simulink model "Group44PACEMAKER"  (R2022b)
settings: Solver=FixedStepAuto  StartTime=0.0  StopTime=4  FixedStep=1e-3  RelTol=1e-3  EnableMultiTasking=on
undefined symbols (not defined in the file): D0, D1, D10, D11, D12, D13, D2, D3, D4, D5, D6, D7, D8, D9, PTA0, PTA1, PTA2, PTB23, PTB9, PTC16, PTC17, PTC2, PTC3, PTC4, PTD0, PTD1, PTD2, PTD3
libraries: frdmk64flib x14
settings Model: PacingRate=0.200000  ExtModeTrigDuration=5  LastModifiedBy=Admin
settings OptimizationCC: EnhancedBackFolding=on  PassReuseOutputArgsAs=Individual arguments  ZeroExternalMemoryAtStartup=off  ZeroInternalMemoryAtStartup=off  MaxStackSize=64  OptimizeBlockOrder=speed  DifferentSizesBufferReuse=on  OptimizationCustomize=off  EfficientTunableParamExpr=on
settings DebuggingCC: ParameterTunabilityLossMsg=error
settings HardwareCC: ProdBitPerPointer=32  ProdBitPerSizeT=32  ProdBitPerPtrDiffT=32  ProdLargestAtomicInteger=Long  ProdLargestAtomicFloat=Double  ProdWordSize=32  ProdHWDeviceType=ARM Compatible->ARM Cortex
settings SFSimCC: MATLABDynamicMemAlloc=off
settings RTWCC: Description=Embedded Coder  SystemTargetFile=ert.tlc  HardwareBoard=NXP FRDM-K64F  TLCOptions="-aInlineSetEventsForThisBaseRateFcn=TLC_FALSE -aSuppressMultiTaskScheduler=TLC_FALSE  -aRateBasedStepFcn=0"  TemplateMakefile=ert_default_tmf  Toolchain=GNU Tools for ARM Embedded Processors
settings CodeAppCC: ForceParamTrailComments=on  IgnoreCustomStorageClasses=off  OperatorAnnotations=on  SimulinkDataObjDesc=on  SFDataObjDesc=on  InsertBlockDesc=on
settings ERTTargetCC: ExtModeTransport=4  ExtModeMexFile=sendToCommService

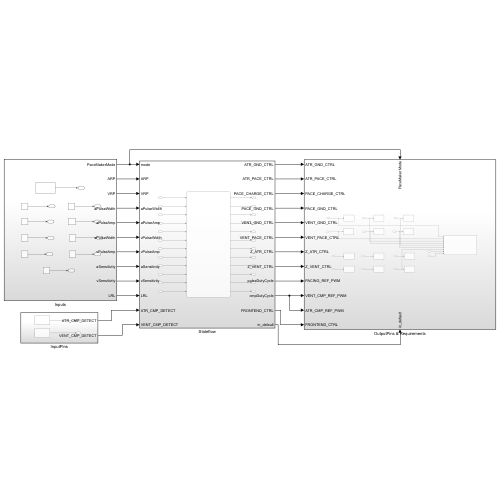
[thumbnail: Simulink's stored preview of the top-level diagram]
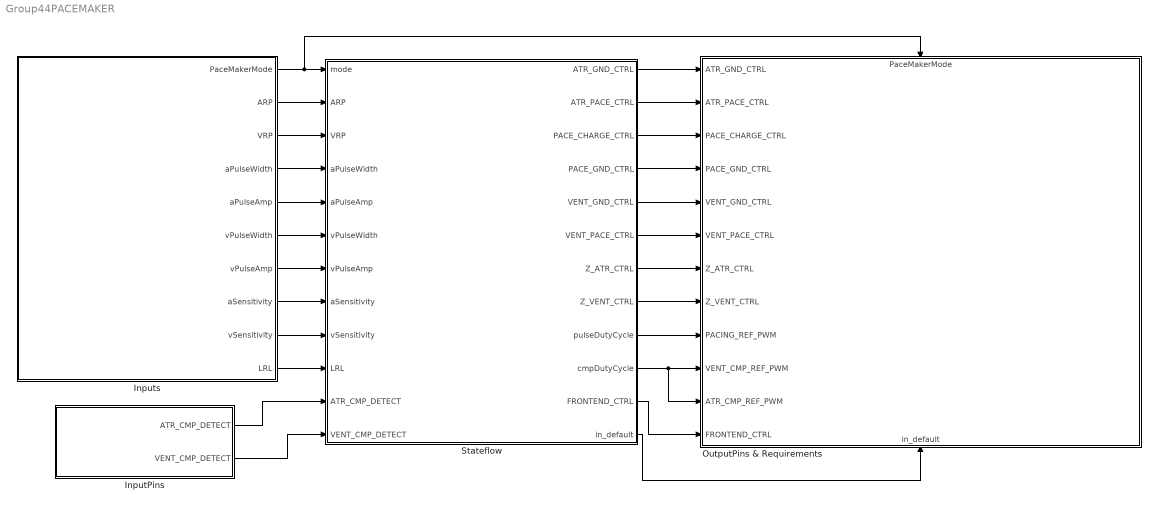
== system Group44PACEMAKER ==
  InputPins : Subsystem
  Inputs : Subsystem
  OutputPins & Requirements : Subsystem
      settings: PortSchema="{\"entries\":[{\"content\":{\"sides\":[{\"content\":{\"connectorIds\":[\"In1\",\"In2\",\"In3\",\"In4\",\"In5\",\"In6\",\"In7\",\"In8\",\"In9\",\"In10\",\"In11\",\"In12\"]},\"type\":\"ConnectorPlacement.EquallySpacedRectSide\",\"uuid\":\"f209b0ac-f79a-4701-a17d-e6e4657793a5\"},{\"content\":{\"connectorIds\":[],\"side\":\"RIGHT\"},\"type\":\"ConnectorPlacement.EquallySpacedRectSide\",\"uuid\":\"7d13a426-91e0-4712-bb01-5d8563f6962a\"},{\"content\":{\"connectorIds\":[\"In13\"],\"side\":\"TOP\"},\"type\":\"ConnectorPlacement.EquallySpacedRectSide\",\"uuid\":\"d5c2df9e-5684-45ec-bc45-fd2dab74cc87\"},{\"content\":{\"connectorIds\":[\"In14\"],\"side\":\"BOTTOM\"},\"type\":\"ConnectorPlacement.EquallySpacedRectSide\",\"uuid\":\"bae969d9-528a-49b4-ab28-7d9f0a0e5f3c\"}]},\"type\":\"ConnectorPlacement.EquallySpacedConnector\",\"uuid\":\"bb7a9bd2-ec42-4c9d-ad79-06266cd920c3\"}],\"packageUris\":[\"http://schema.mathworks.com/mf0/Connector/R2020b\"],\"version\":\"1.0\"}"
  Stateflow : Subsystem
  wires:
  Inputs/2(ARP) -> Stateflow/2(ARP)
  Inputs/3(VRP) -> Stateflow/3(VRP)
  Inputs/4(aPulseWidth) -> Stateflow/4(aPulseWidth)
  Inputs/6(vPulseWidth) -> Stateflow/6(vPulseWidth)
  Inputs/5(aPulseAmp) -> Stateflow/5(aPulseAmp)
  Inputs/7(vPulseAmp) -> Stateflow/7(vPulseAmp)
  Inputs/9(vSensitivity) -> Stateflow/9(vSensitivity)
  Inputs/8(aSensitivity) -> Stateflow/8(aSensitivity)
  Inputs/10(LRL) -> Stateflow/10(LRL)
  Inputs/1(PaceMakerMode) -> OutputPins & Requirements/13(PaceMakerMode), Stateflow/1(mode)
  InputPins/1(ATR_CMP_DETECT) -> Stateflow/11(ATR_CMP_DETECT)
  InputPins/2(VENT_CMP_DETECT) -> Stateflow/12(VENT_CMP_DETECT)
  Stateflow/1(ATR_GND_CTRL) -> OutputPins & Requirements/1(ATR_GND_CTRL)
  Stateflow/2(ATR_PACE_CTRL) -> OutputPins & Requirements/2(ATR_PACE_CTRL)
  Stateflow/3(PACE_CHARGE_CTRL) -> OutputPins & Requirements/3(PACE_CHARGE_CTRL)
  Stateflow/4(PACE_GND_CTRL) -> OutputPins & Requirements/4(PACE_GND_CTRL)
  Stateflow/5(VENT_GND_CTRL) -> OutputPins & Requirements/5(VENT_GND_CTRL)
  Stateflow/6(VENT_PACE_CTRL) -> OutputPins & Requirements/6(VENT_PACE_CTRL)
  Stateflow/7(Z_ATR_CTRL) -> OutputPins & Requirements/7(Z_ATR_CTRL)
  Stateflow/8(Z_VENT_CTRL) -> OutputPins & Requirements/8(Z_VENT_CTRL)
  Stateflow/9(pulseDutyCycle) -> OutputPins & Requirements/9(PACING_REF_PWM)
  Stateflow/10(cmpDutyCycle) -> OutputPins & Requirements/11(ATR_CMP_REF_PWM), OutputPins & Requirements/10(VENT_CMP_REF_PWM)
  Stateflow/11(FRONTEND_CTRL) -> OutputPins & Requirements/12(FRONTEND_CTRL)
  Stateflow/12(in_default) -> OutputPins & Requirements/14(in_default)

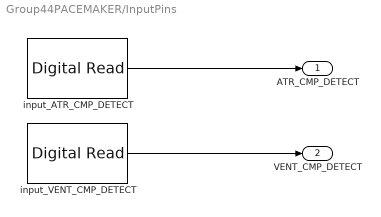
== system Group44PACEMAKER/InputPins ==
  input_ATR_CMP_DETECT : frdmk64flib/Digital Read  Whichpin=PTC16 (D0)  SampleTime=-1
  input_VENT_CMP_DETECT : frdmk64flib/Digital Read  Whichpin=PTC17 (D1)  SampleTime=-1
  ATR_CMP_DETECT : Outport  OutDataTypeStr=boolean
  VENT_CMP_DETECT : Outport  Port=2  OutDataTypeStr=boolean
  wires:
  input_ATR_CMP_DETECT/1 -> ATR_CMP_DETECT/1
  input_VENT_CMP_DETECT/1 -> VENT_CMP_DETECT/1

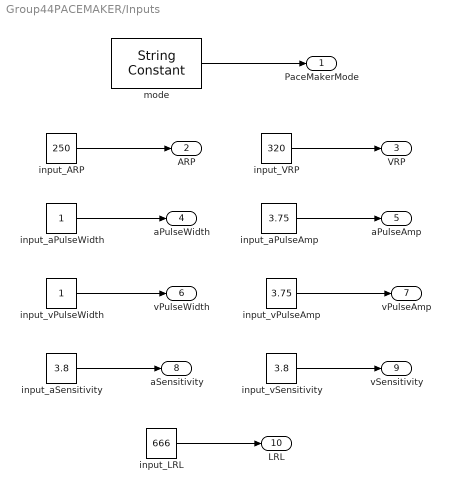
== system Group44PACEMAKER/Inputs ==
  input_ARP : Constant  Value=250  OutDataTypeStr=double
  input_LRL : Constant  Value=666  OutDataTypeStr=double
  input_VRP : Constant  Value=320  OutDataTypeStr=double
  input_aPulseAmp : Constant  Value=3.75  OutDataTypeStr=double
  input_aPulseWidth : Constant  OutDataTypeStr=double
  input_aSensitivity : Constant  Value=3.8  OutDataTypeStr=double
  input_vPulseAmp : Constant  Value=3.75  OutDataTypeStr=double
  input_vPulseWidth : Constant  OutDataTypeStr=double
  input_vSensitivity : Constant  Value=3.8  OutDataTypeStr=double
  mode : StringConstant  String="\"AOO\""
  PaceMakerMode : Outport  OutDataTypeStr=string
  ARP : Outport  Port=2  OutDataTypeStr=double  Unit=msec
  VRP : Outport  Port=3  OutDataTypeStr=double  Unit=msec
  aPulseWidth : Outport  Port=4  OutDataTypeStr=double  Unit=msec
  aPulseAmp : Outport  Port=5  OutDataTypeStr=double  Unit=V
  vPulseWidth : Outport  Port=6  OutDataTypeStr=double  Unit=msec
  vPulseAmp : Outport  Port=7  OutDataTypeStr=double  Unit=V
  aSensitivity : Outport  Port=8  OutDataTypeStr=double  Unit=V
  vSensitivity : Outport  Port=9  OutDataTypeStr=double  Unit=V
  LRL : Outport  Port=10  OutDataTypeStr=double  Unit=msec
  wires:
  mode/1 -> PaceMakerMode/1
  input_aPulseAmp/1 -> aPulseAmp/1
  input_ARP/1 -> ARP/1
  input_VRP/1 -> VRP/1
  input_aPulseWidth/1 -> aPulseWidth/1
  input_vPulseWidth/1 -> vPulseWidth/1
  input_vPulseAmp/1 -> vPulseAmp/1
  input_vSensitivity/1 -> vSensitivity/1
  input_aSensitivity/1 -> aSensitivity/1
  input_LRL/1 -> LRL/1

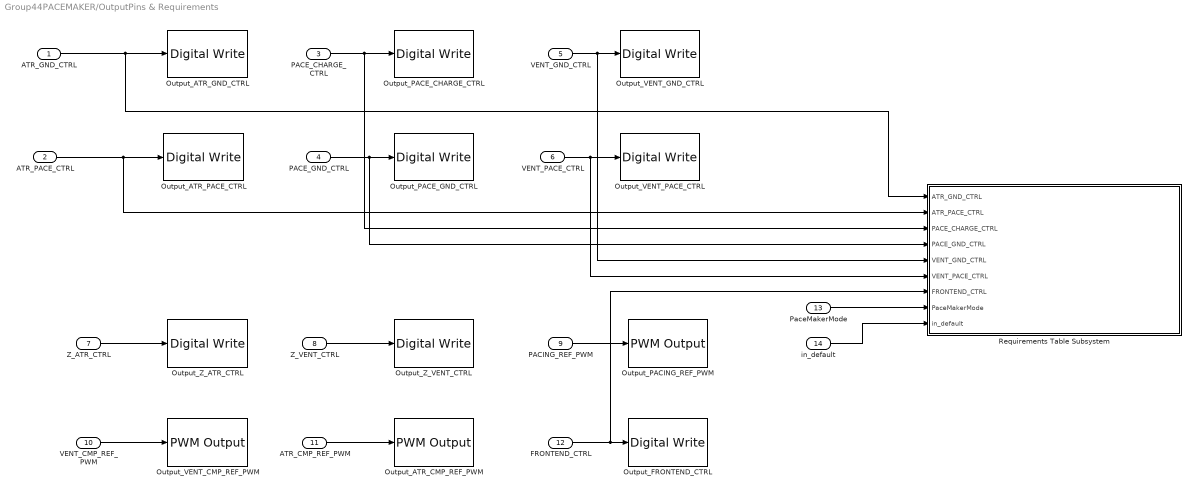
== system Group44PACEMAKER/OutputPins & Requirements ==
  ATR_GND_CTRL : Inport  OutDataTypeStr=boolean
  ATR_PACE_CTRL : Inport  Port=2  OutDataTypeStr=boolean
  PACE_CHARGE_CTRL : Inport  Port=3  OutDataTypeStr=boolean
  PACE_GND_CTRL : Inport  Port=4  OutDataTypeStr=boolean
  VENT_GND_CTRL : Inport  Port=5  OutDataTypeStr=boolean
  VENT_PACE_CTRL : Inport  Port=6  OutDataTypeStr=boolean
  Z_ATR_CTRL : Inport  Port=7  OutDataTypeStr=boolean
  Z_VENT_CTRL : Inport  Port=8  OutDataTypeStr=boolean
  PACING_REF_PWM : Inport  Port=9  OutDataTypeStr=double
  VENT_CMP_REF_PWM : Inport  Port=10  OutDataTypeStr=double
  ATR_CMP_REF_PWM : Inport  Port=11  OutDataTypeStr=double
  FRONTEND_CTRL : Inport  Port=12  OutDataTypeStr=boolean
  PaceMakerMode : Inport  Port=13  OutDataTypeStr=string
  in_default : Inport  Port=14  OutDataTypeStr=boolean
  Output_ATR_CMP_REF_PWM : frdmk64flib/PWM Output  Whichpin=PTC2 (D6)  InitialFrequency=2000  InitialDutyCycle=0
  Output_ATR_GND_CTRL : frdmk64flib/Digital Write  Whichpin=PTD2 (D11)
  Output_ATR_PACE_CTRL : frdmk64flib/Digital Write  Whichpin=PTA0 (D8)
  Output_FRONTEND_CTRL : frdmk64flib/Digital Write  Whichpin=PTD1 (D13)
  Output_PACE_CHARGE_CTRL : frdmk64flib/Digital Write  Whichpin=PTB9 (D2)
  Output_PACE_GND_CTRL : frdmk64flib/Digital Write  Whichpin=PTD0 (D10)
  Output_PACING_REF_PWM : frdmk64flib/PWM Output  Whichpin=PTA2 (D5)  InitialFrequency=2000  InitialDutyCycle=0
  Output_VENT_CMP_REF_PWM : frdmk64flib/PWM Output  Whichpin=PTA1 (D3)  InitialFrequency=2000  InitialDutyCycle=0
  Output_VENT_GND_CTRL : frdmk64flib/Digital Write  Whichpin=PTD3 (D12)
  Output_VENT_PACE_CTRL : frdmk64flib/Digital Write  Whichpin=PTC4 (D9)
  Output_Z_ATR_CTRL : frdmk64flib/Digital Write  Whichpin=PTB23 (D4)
  Output_Z_VENT_CTRL : frdmk64flib/Digital Write  Whichpin=PTC3 (D7)
  Requirements Table Subsystem : Subsystem
  wires:
  ATR_GND_CTRL/1 -> Requirements Table Subsystem/1(ATR_GND_CTRL), Output_ATR_GND_CTRL/1
  PACE_CHARGE_CTRL/1 -> Requirements Table Subsystem/3(PACE_CHARGE_CTRL), Output_PACE_CHARGE_CTRL/1
  VENT_GND_CTRL/1 -> Requirements Table Subsystem/5(VENT_GND_CTRL), Output_VENT_GND_CTRL/1
  VENT_PACE_CTRL/1 -> Requirements Table Subsystem/6(VENT_PACE_CTRL), Output_VENT_PACE_CTRL/1
  PACE_GND_CTRL/1 -> Requirements Table Subsystem/4(PACE_GND_CTRL), Output_PACE_GND_CTRL/1
  ATR_PACE_CTRL/1 -> Requirements Table Subsystem/2(ATR_PACE_CTRL), Output_ATR_PACE_CTRL/1
  Z_ATR_CTRL/1 -> Output_Z_ATR_CTRL/1
  Z_VENT_CTRL/1 -> Output_Z_VENT_CTRL/1
  PACING_REF_PWM/1 -> Output_PACING_REF_PWM/1
  ATR_CMP_REF_PWM/1 -> Output_ATR_CMP_REF_PWM/1
  VENT_CMP_REF_PWM/1 -> Output_VENT_CMP_REF_PWM/1
  FRONTEND_CTRL/1 -> Output_FRONTEND_CTRL/1, Requirements Table Subsystem/7(FRONTEND_CTRL)
  PaceMakerMode/1 -> Requirements Table Subsystem/8(PaceMakerMode)
  in_default/1 -> Requirements Table Subsystem/9(in_default)

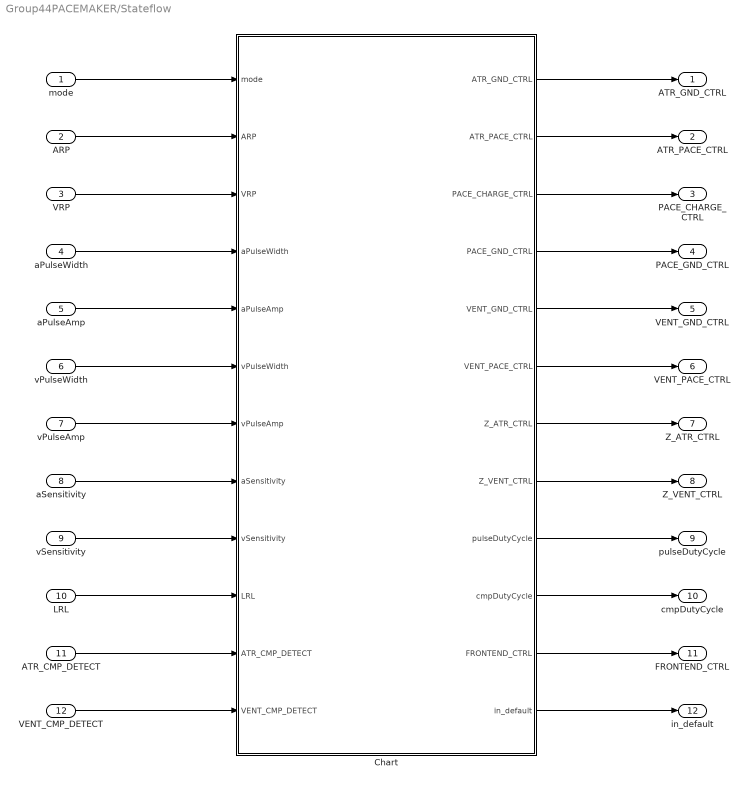
== system Group44PACEMAKER/Stateflow ==
  mode : Inport  OutDataTypeStr=string
  ARP : Inport  Port=2  OutDataTypeStr=double  Unit=msec
  VRP : Inport  Port=3  OutDataTypeStr=double  Unit=msec
  aPulseWidth : Inport  Port=4  OutDataTypeStr=double  Unit=msec
  aPulseAmp : Inport  Port=5  OutDataTypeStr=double  Unit=V
  vPulseWidth : Inport  Port=6  OutDataTypeStr=double  Unit=msec
  vPulseAmp : Inport  Port=7  OutDataTypeStr=double  Unit=V
  aSensitivity : Inport  Port=8  OutDataTypeStr=double  Unit=V
  vSensitivity : Inport  Port=9  OutDataTypeStr=double  Unit=V
  LRL : Inport  Port=10  OutDataTypeStr=double  Unit=msec
  ATR_CMP_DETECT : Inport  Port=11  OutDataTypeStr=boolean
  VENT_CMP_DETECT : Inport  Port=12  OutDataTypeStr=boolean
  Chart : Stateflow chart  TreatAsAtomicUnit=on
      settings: PortSchema="{\"entries\":[{\"content\":{\"sides\":[{\"content\":{\"connectorIds\":[\"In8\",\"In1\",\"In2\",\"In3\",\"In9\",\"In5\",\"In10\",\"In12\",\"In11\",\"In4\",\"In6\",\"In7\"]},\"type\":\"ConnectorPlacement.EquallySpacedRectSide\",\"uuid\":\"55977362-650a-4bd6-88e9-af7768e99957\"},{\"content\":{\"connectorIds\":[\"Out1\",\"Out2\",\"Out3\",\"Out4\",\"Out5\",\"Out6\",\"Out7\",\"Out8\",\"Out9\",\"Out10\",\"Out11\",\"Out12\"],\"side\":\"RIGHT\"},\"type\":\"ConnectorPlacement.EquallySpacedRectSide\",\"uuid\":\"ff06bc7e-4f3c-429f-a92b-8b0b296c3971\"},{\"content\":{\"connectorIds\":[],\"side\":\"TOP\"},\"type\":\"ConnectorPlacement.EquallySpacedRectSide\",\"uuid\":\"055d3fa4-5ac7-41a2-af91-00b36b97cf6e\"}]},\"type\":\"ConnectorPlacement.EquallySpacedConnector\",\"uuid\":\"4b7bf5c6-9d02-4e0c-984a-6477d477a142\"}],\"packageUris\":[\"http://schema.mathworks.com/mf0/Connector/R2020b\"],\"version\":\"1.0\"}"
  ATR_GND_CTRL : Outport  OutDataTypeStr=boolean
  ATR_PACE_CTRL : Outport  Port=2  OutDataTypeStr=boolean
  PACE_CHARGE_CTRL : Outport  Port=3  OutDataTypeStr=boolean
  PACE_GND_CTRL : Outport  Port=4  OutDataTypeStr=boolean
  VENT_GND_CTRL : Outport  Port=5  OutDataTypeStr=boolean
  VENT_PACE_CTRL : Outport  Port=6  OutDataTypeStr=boolean
  Z_ATR_CTRL : Outport  Port=7  OutDataTypeStr=boolean
  Z_VENT_CTRL : Outport  Port=8  OutDataTypeStr=boolean
  pulseDutyCycle : Outport  Port=9  OutDataTypeStr=double
  cmpDutyCycle : Outport  Port=10  OutDataTypeStr=double
  FRONTEND_CTRL : Outport  Port=11  OutDataTypeStr=boolean
  in_default : Outport  Port=12  OutDataTypeStr=boolean
  wires:
  ARP/1 -> Chart/1(ARP)
  VRP/1 -> Chart/2(VRP)
  aPulseWidth/1 -> Chart/3(aPulseWidth)
  LRL/1 -> Chart/4(LRL)
  vPulseWidth/1 -> Chart/5(vPulseWidth)
  ATR_CMP_DETECT/1 -> Chart/6(ATR_CMP_DETECT)
  VENT_CMP_DETECT/1 -> Chart/7(VENT_CMP_DETECT)
  mode/1 -> Chart/8(mode)
  aPulseAmp/1 -> Chart/9(aPulseAmp)
  vPulseAmp/1 -> Chart/10(vPulseAmp)
  vSensitivity/1 -> Chart/11(vSensitivity)
  aSensitivity/1 -> Chart/12(aSensitivity)
  Chart/10(cmpDutyCycle) -> cmpDutyCycle/1
  Chart/9(pulseDutyCycle) -> pulseDutyCycle/1
  Chart/8(Z_VENT_CTRL) -> Z_VENT_CTRL/1
  Chart/7(Z_ATR_CTRL) -> Z_ATR_CTRL/1
  Chart/6(VENT_PACE_CTRL) -> VENT_PACE_CTRL/1
  Chart/5(VENT_GND_CTRL) -> VENT_GND_CTRL/1
  Chart/4(PACE_GND_CTRL) -> PACE_GND_CTRL/1
  Chart/3(PACE_CHARGE_CTRL) -> PACE_CHARGE_CTRL/1
  Chart/2(ATR_PACE_CTRL) -> ATR_PACE_CTRL/1
  Chart/1(ATR_GND_CTRL) -> ATR_GND_CTRL/1
  Chart/11(FRONTEND_CTRL) -> FRONTEND_CTRL/1
  Chart/12(in_default) -> in_default/1

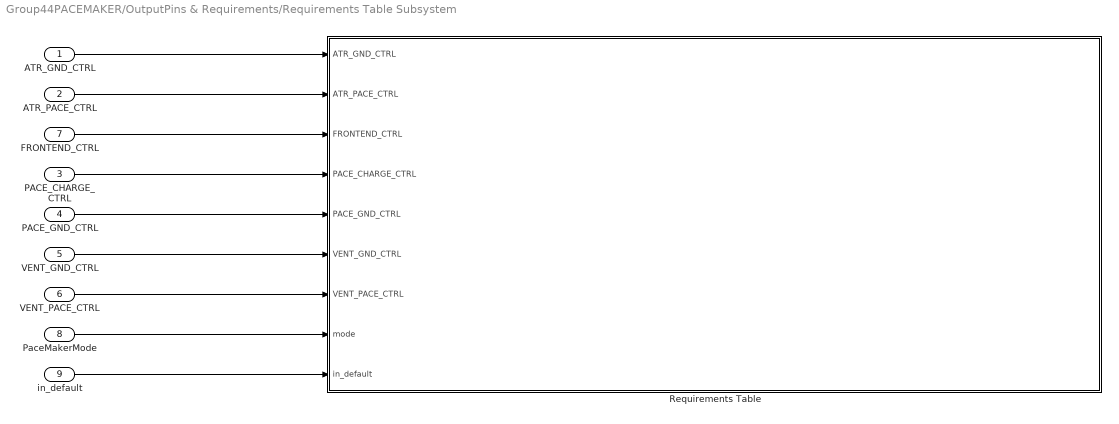
== system Group44PACEMAKER/OutputPins & Requirements/Requirements Table Subsystem ==
  ATR_GND_CTRL : Inport  OutDataTypeStr=boolean
  ATR_PACE_CTRL : Inport  Port=2  OutDataTypeStr=boolean
  PACE_CHARGE_CTRL : Inport  Port=3  OutDataTypeStr=boolean
  PACE_GND_CTRL : Inport  Port=4  OutDataTypeStr=boolean
  VENT_GND_CTRL : Inport  Port=5  OutDataTypeStr=boolean
  VENT_PACE_CTRL : Inport  Port=6  OutDataTypeStr=boolean
  FRONTEND_CTRL : Inport  Port=7  OutDataTypeStr=boolean
  PaceMakerMode : Inport  Port=8  OutDataTypeStr=string
  in_default : Inport  Port=9  OutDataTypeStr=boolean
  Requirements Table : Requirements Table  TreatAsAtomicUnit=on
  wires:
  ATR_GND_CTRL/1 -> Requirements Table/1(ATR_GND_CTRL)
  ATR_PACE_CTRL/1 -> Requirements Table/2(ATR_PACE_CTRL)
  PACE_CHARGE_CTRL/1 -> Requirements Table/4(PACE_CHARGE_CTRL)
  PACE_GND_CTRL/1 -> Requirements Table/5(PACE_GND_CTRL)
  VENT_GND_CTRL/1 -> Requirements Table/6(VENT_GND_CTRL)
  VENT_PACE_CTRL/1 -> Requirements Table/7(VENT_PACE_CTRL)
  FRONTEND_CTRL/1 -> Requirements Table/3(FRONTEND_CTRL)
  PaceMakerMode/1 -> Requirements Table/8(mode)
  in_default/1 -> Requirements Table/9(in_default)

== stateflow chart Group44PACEMAKER/OutputPins & Requirements/Requirements Table Subsystem/Requirements Table ==
  (default) -> (junction 1073742542)
  (junction 1073742542) -> (junction 1073742543) : {
      | % SF_REQ_REV_07
      | }
  (junction 1073742543) -> (junction 1073742545) : {
      | % HEADER_ASSIGNMENTS
      |
      | }
  (junction 1073742545) -> (junction 1073742547) : {
      | % START_A_4
      | }
  (junction 1073742547) -> (junction 1073742549) : {
      | }
  (junction 1073742549) -> (junction 1073742551) : {
      | reqtable_assumption((t>=0), 4);
      | }
  (junction 1073742551) -> (junction 1073742553) : {
      | }
  (junction 1073742553) -> (junction 1073742555) : {
      | % END_A_4
      | }
  (junction 1073742555) -> (junction 1073742557) : {
      | % START_R_28
      | }
  (junction 1073742557) -> (junction 1073742559) : {
      | }
  (junction 1073742559) -> (junction 1073742561)
  (junction 1073742561) -> (junction 1073742563) [order 1] : [(((in_default) == (1))) && (((PACE_CHARGE_CTRL ) == (0)))]
  (junction 1073742561) -> (junction 1073742569) [order 2]
  (junction 1073742563) -> (junction 1073742565) : {
      | reqtable_postcondition((((ATR_PACE_CTRL ) == (0))) && (((VENT_PACE_CTRL ) == (0))) && (((ATR_GND_CTRL ) == (0))) && (((VENT_GND_CTRL ) == (0))) && (((PACE_GND_CTRL) == (0))), 'R:1');
      |
      |
      | }
  (junction 1073742565) -> (junction 1073742567) : {
      | }
  (junction 1073742567) -> (junction 1073742569)
  (junction 1073742569) -> (junction 1073742571)
  (junction 1073742571) -> (junction 1073742573) : {
      | % END_R_28
      | }
  (junction 1073742573) -> (junction 1073742575) : {
      | % START_R_1
      | }
  (junction 1073742575) -> (junction 1073742577) : {
      | }
  (junction 1073742577) -> (junction 1073742579)
  (junction 1073742579) -> (junction 1073742581) [order 1] : [(((in_default) == (0))) && (((PACE_CHARGE_CTRL ) == (1))) && (mode == "AOO" || mode == "AAI")]
  (junction 1073742579) -> (junction 1073742587) [order 2]
  (junction 1073742581) -> (junction 1073742583) : {
      | reqtable_postcondition((((ATR_PACE_CTRL ) == (0))) && (((VENT_PACE_CTRL ) == (0))) && (((ATR_GND_CTRL ) == (1))) && (((VENT_GND_CTRL ) == (0))) && (((PACE_GND_CTRL) == (1))), 'R:2');
      |
      |
      | }
  (junction 1073742583) -> (junction 1073742585) : {
      | }
  (junction 1073742585) -> (junction 1073742587)
  (junction 1073742587) -> (junction 1073742589)
  (junction 1073742589) -> (junction 1073742591) : {
      | % END_R_1
      | }
  (junction 1073742591) -> (junction 1073742593) : {
      | % START_R_25
      | }
  (junction 1073742593) -> (junction 1073742595) : {
      | }
  (junction 1073742595) -> (junction 1073742597)
  (junction 1073742597) -> (junction 1073742599) [order 1] : [(((in_default) == (0))) && (((PACE_CHARGE_CTRL ) == (1))) && (mode == "VOO" || mode == "VVI")]
  (junction 1073742597) -> (junction 1073742605) [order 2]
  (junction 1073742599) -> (junction 1073742601) : {
      | reqtable_postcondition((((ATR_PACE_CTRL ) == (0))) && (((VENT_PACE_CTRL ) == (0))) && (((ATR_GND_CTRL ) == (0))) && (((VENT_GND_CTRL ) == (1))) && (((PACE_GND_CTRL) == (1))), 'R:3');
      |
      |
      | }
  (junction 1073742601) -> (junction 1073742603) : {
      | }
  (junction 1073742603) -> (junction 1073742605)
  (junction 1073742605) -> (junction 1073742607)
  (junction 1073742607) -> (junction 1073742609) : {
      | % END_R_25
      | }
  (junction 1073742609) -> (junction 1073742611) : {
      | % START_R_10
      | }
  (junction 1073742611) -> (junction 1073742613) : {
      | }
  (junction 1073742613) -> (junction 1073742615)
  (junction 1073742615) -> (junction 1073742617) [order 1] : [(((in_default) == (0))) && (((PACE_CHARGE_CTRL ) == (0))) && (mode == "AOO" || mode == "AAI")]
  (junction 1073742615) -> (junction 1073742623) [order 2]
  (junction 1073742617) -> (junction 1073742619) : {
      | reqtable_postcondition((((ATR_PACE_CTRL ) == (1))) && (((VENT_PACE_CTRL ) == (0))) && (((ATR_GND_CTRL ) == (0))) && (((VENT_GND_CTRL ) == (0))) && (((PACE_GND_CTRL) == (1))), 'R:4');
      |
      |
      | }
  (junction 1073742619) -> (junction 1073742621) : {
      | }
  (junction 1073742621) -> (junction 1073742623)
  (junction 1073742623) -> (junction 1073742625)
  (junction 1073742625) -> (junction 1073742627) : {
      | % END_R_10
      | }
  (junction 1073742627) -> (junction 1073742629) : {
      | % START_R_19
      | }
  (junction 1073742629) -> (junction 1073742631) : {
      | }
  (junction 1073742631) -> (junction 1073742633)
  (junction 1073742633) -> (junction 1073742635) [order 1] : [(((in_default) == (0))) && (((PACE_CHARGE_CTRL ) == (0))) && (mode == "VOO" || mode == "VVI")]
  (junction 1073742633) -> (junction 1073742641) [order 2]
  (junction 1073742635) -> (junction 1073742637) : {
      | reqtable_postcondition((((ATR_PACE_CTRL ) == (0))) && (((VENT_PACE_CTRL ) == (1))) && (((ATR_GND_CTRL ) == (0))) && (((VENT_GND_CTRL ) == (0))) && (((PACE_GND_CTRL) == (1))), 'R:5');
      |
      |
      | }
  (junction 1073742637) -> (junction 1073742639) : {
      | }
  (junction 1073742639) -> (junction 1073742641)
  (junction 1073742641) -> (junction 1073742643)
  (junction 1073742643) -> (junction 1073742645) : {
      | % END_R_19
      | }
  (junction 1073742645) -> (junction 1073742647) : {
      | % START_R_13
      | }
  (junction 1073742647) -> (junction 1073742649) : {
      | }
  (junction 1073742649) -> (junction 1073742651)
  (junction 1073742651) -> (junction 1073742653) [order 1] : [(((in_default) == (0))) && (((FRONTEND_CTRL ) == (1))) && (mode == "AAI" || mode == "VVI")]
  (junction 1073742651) -> (junction 1073742659) [order 2]
  (junction 1073742653) -> (junction 1073742655) : {
      | reqtable_postcondition((((ATR_PACE_CTRL ) == (0))) && (((VENT_PACE_CTRL ) == (0))) && (((PACE_GND_CTRL) == (1))), 'R:6');
      |
      |
      | }
  (junction 1073742655) -> (junction 1073742657) : {
      | }
  (junction 1073742657) -> (junction 1073742659)
  (junction 1073742659) -> (junction 1073742661)
  (junction 1073742661) -> (junction 1073742663) : {
      | % END_R_13
      | }
  data: ATR_GND_CTRL input boolean; ATR_PACE_CTRL input boolean; FRONTEND_CTRL input boolean; PACE_CHARGE_CTRL input boolean; PACE_GND_CTRL input boolean; VENT_GND_CTRL input boolean; VENT_PACE_CTRL input boolean; mode input string; in_default input boolean

== stateflow chart Group44PACEMAKER/Stateflow/Chart ==
  state PaceAtria
    entry:
    PACE_CHARGE_CTRL = false;
    PACE_GND_CTRL = true;
    ATR_PACE_CTRL = true;
    ATR_GND_CTRL = false;
    Z_ATR_CTRL = false;
    Z_VENT_CTRL = false;
    VENT_GND_CTRL = false;
    VENT_PACE_CTRL = false;
  state PaceVentricle
    entry:
    PACE_CHARGE_CTRL = false;
    PACE_GND_CTRL = true;
    ATR_PACE_CTRL = false;
    ATR_GND_CTRL = false;
    Z_ATR_CTRL = false;
    Z_VENT_CTRL = false;
    VENT_GND_CTRL = false;
    VENT_PACE_CTRL = true;
  state ChargeC22_Atrial_DischargeC21
    entry:
    ATR_PACE_CTRL = false;
    VENT_PACE_CTRL = false;
    PACE_CHARGE_CTRL = true;
    PACE_GND_CTRL = true;
    Z_ATR_CTRL = false;
    Z_VENT_CTRL = false;
    ATR_GND_CTRL = true;
    VENT_GND_CTRL = false;
  state ChargeC22_Ventricular_DischargeC21
    entry:
    ATR_PACE_CTRL = false;
    VENT_PACE_CTRL = false;
    PACE_CHARGE_CTRL = true;
    PACE_GND_CTRL = true;
    Z_ATR_CTRL = false;
    Z_VENT_CTRL = false;
    ATR_GND_CTRL = false;
    VENT_GND_CTRL = true;
  state AtrialAlertPeriod
    FRONTEND_CTRL = true;
  state VentricularAlertPeriod
    FRONTEND_CTRL = true;
  state Default_Starting_State
    entry:
    in_default = true;
  PaceAtria -> ChargeC22_Atrial_DischargeC21 [order 1] : after(aPulseWidth,msec)[mode=="AOO"]
  PaceVentricle -> ChargeC22_Ventricular_DischargeC21 [order 1] : after(vPulseWidth,msec)[mode=="VOO"]
  ChargeC22_Atrial_DischargeC21 -> PaceAtria [order 1] : after(LRL-aPulseWidth,msec)[mode=="AOO"]
  PaceAtria -> ChargeC22_Atrial_DischargeC21 [order 2] : after(aPulseWidth,msec)[mode=="AAI"]
  AtrialAlertPeriod -> PaceAtria [order 2] : after(LRL-ARP-aPulseWidth,msec){FRONTEND_CTRL=false}
  ChargeC22_Ventricular_DischargeC21 -> PaceVentricle [order 1] : after(LRL-vPulseWidth,msec)[mode=="VOO"]
  PaceVentricle -> ChargeC22_Ventricular_DischargeC21 [order 2] : after(vPulseWidth,msec)[mode=="VVI"]
  VentricularAlertPeriod -> PaceVentricle [order 2] : after(LRL-VRP-vPulseWidth,msec){FRONTEND_CTRL=false}
  ChargeC22_Atrial_DischargeC21 -> AtrialAlertPeriod [order 2] : after(ARP,msec)[mode=="AAI"]
  VentricularAlertPeriod -> ChargeC22_Ventricular_DischargeC21 [order 1] : [VENT_CMP_DETECT == true ]
  AtrialAlertPeriod -> ChargeC22_Atrial_DischargeC21 [order 1] : [ATR_CMP_DETECT == true ]
  ChargeC22_Ventricular_DischargeC21 -> VentricularAlertPeriod [order 2] : after(VRP,msec)[mode=="VVI"]
  (junction 103) -> ChargeC22_Atrial_DischargeC21 [order 2] : [mode=="AAI"]{cmpDutyCycle=aSensitivity/5.0*100}
  (junction 103) -> ChargeC22_Atrial_DischargeC21 [order 1] : [mode=="AOO"]
  (junction 105) -> ChargeC22_Ventricular_DischargeC21 [order 1] : [mode=="VOO"]
  (junction 105) -> ChargeC22_Ventricular_DischargeC21 [order 2] : [mode=="VVI"]{cmpDutyCycle=vSensitivity/5.0*100}
  (junction 59) -> (junction 103) [order 1] : after(aPulseWidth,msec)[mode=="AOO"||mode=="AAI"]{pulseDutyCycle=aPulseAmp/5.0*100}
  (junction 59) -> (junction 105) [order 2] : after(vPulseWidth,msec)[mode=="VOO"||mode=="VVI"]{pulseDutyCycle=vPulseAmp/5.0*100}
  Default_Starting_State -> (junction 59) : {in_default = false}
  (default) -> Default_Starting_State
  data: ARP input double; VRP input double; aPulseWidth input double; LRL input double; vPulseWidth input double; ATR_GND_CTRL output boolean; ATR_PACE_CTRL output boolean; PACE_CHARGE_CTRL output boolean; PACE_GND_CTRL output boolean; VENT_GND_CTRL output boolean; VENT_PACE_CTRL output boolean; Z_ATR_CTRL output boolean; Z_VENT_CTRL output boolean; ATR_CMP_DETECT input boolean; VENT_CMP_DETECT input boolean; mode input string; aPulseAmp input double; vPulseAmp input double; pulseDutyCycle output double; cmpDutyCycle output double; vSensitivity input double; aSensitivity input double; FRONTEND_CTRL output boolean; in_default output boolean
